simulink subsystem "PieroControladoV"  (R2023b)
settings: Solver=VariableStepAuto  StartTime=0.0  StopTime=10.0  RelTol=1e-3
settings Model: Creator=Andrés  LastModifiedBy=Andrés

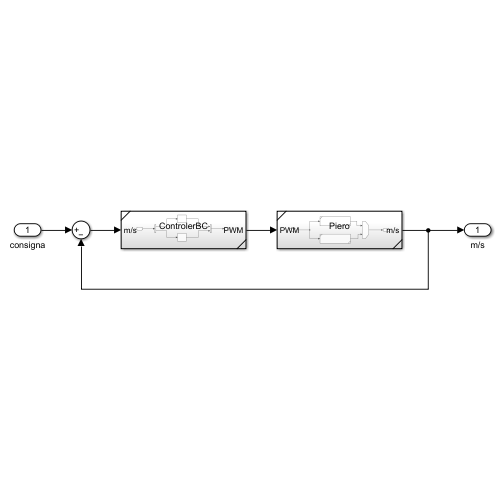
[thumbnail: Simulink's stored preview of the top-level diagram]
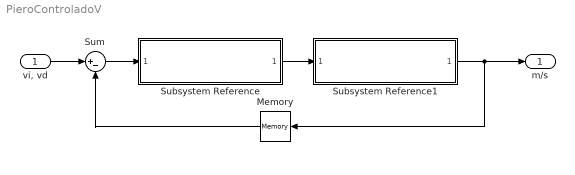
== system PieroControladoV ==
  "vi, vd" : Inport
  Memory : Memory
  Subsystem Reference : Subsystem  ReferencedSubsystem=ControlerBC
  Subsystem Reference1 : Subsystem  ReferencedSubsystem=Piero
  Sum : Sum  Inputs=|+-
  m/s : Outport
  wires:
  Subsystem Reference1/1 -> Memory/1, m/s/1
  Subsystem Reference/1 -> Subsystem Reference1/1
  "vi, vd"/1 -> Sum/1
  Sum/1 -> Subsystem Reference/1
  Memory/1 -> Sum/2
